simulink model "fermentation_dynamic_model_update"  (R2018a)
settings: Solver=VariableStepAuto  StartTime=0.0  StopTime=160  RelTol=1e-3
values from neighbouring files (symbols this model uses):
  ABV_lim = 0.0433    [fermentation_config_update.m]
  E_0 = 0    [fermentation_config_update.m]
  E_mol_mass = 0.04607    [fermentation_config_update.m]
  G_0 = 12.61/142.3*sum_sugars/0.180156    (= 104.992339972)    [fermentation_config_update.m]
  Kb = 10    [fermentation_config_update.m]
  Kd = 0    [fermentation_config_update.m]
  Ki = 0.1    [fermentation_config_update.m]
  Kp = 1.8    [fermentation_config_update.m]
  M_0 = 13.692/142.3*sum_sugars/0.3423    (= 60)    [fermentation_config_update.m]
  N = 0    [fermentation_config_update.m]
  N_0 = 116.205/143.2*sum_sugars/0.504437    (= 343.376857703)    [fermentation_config_update.m]
  p_KG = polyfit(T,K_G,1)    [fermentation_config_update.m]
  p_KiG = polyfit(T,Ki_G,1)    [fermentation_config_update.m]
  p_KiM = polyfit(T,Ki_M,1)    [fermentation_config_update.m]
  p_KM = polyfit(T,K_M,1)    [fermentation_config_update.m]
  p_KN = polyfit(T,K_N,1)    [fermentation_config_update.m]
  p_VG = polyfit(T,V_G,1)    [fermentation_config_update.m]
  p_VM = polyfit(T,V_M,1)    [fermentation_config_update.m]
  p_VN = polyfit(T,V_N,1)    [fermentation_config_update.m]
  R_EG = 1.92    [fermentation_config_update.m]
  R_EM = 3.84    [fermentation_config_update.m]
  R_EN = 5.76    [fermentation_config_update.m]
  R_XG = 0.134    [fermentation_config_update.m]
  R_XM = 0.268    [fermentation_config_update.m]
  R_XN = 0.402    [fermentation_config_update.m]
  T_0 = 12    [fermentation_config_update.m]
  T_c = 12    [fermentation_config_update.m]
  T_s = 12    [fermentation_config_update.m]
  X_0 = 200    [fermentation_config_update.m]
settings Model: Creator=Oscar  LastModifiedBy=Oscar

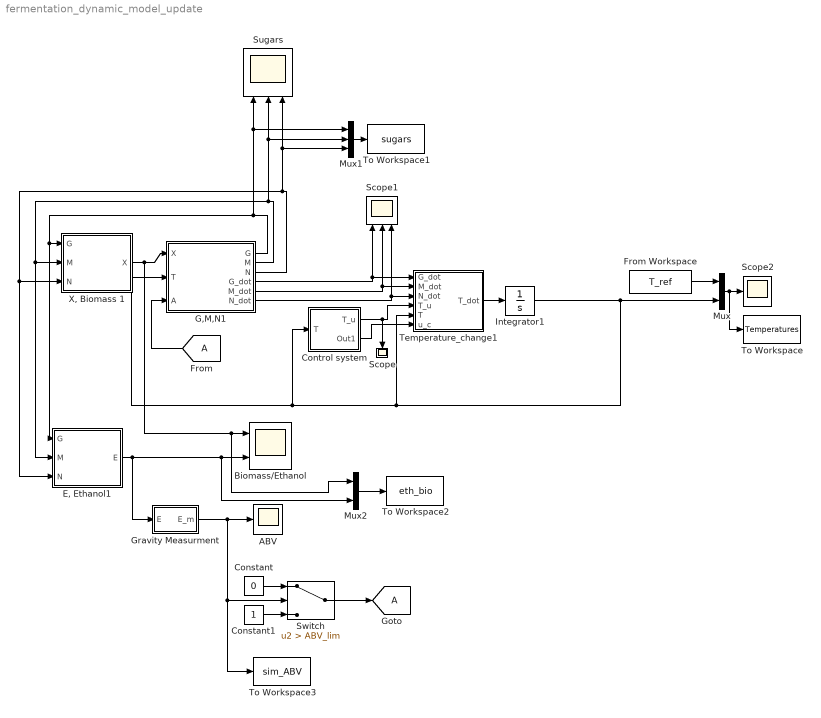
== system fermentation_dynamic_model_update ==
  ABV : Scope
  Biomass/Ethanol : Scope  NumInputPorts=2
  Constant : Constant  Value=0
  Constant1 : Constant
  Control system : Subsystem
  "E, Ethanol1" : Subsystem
  From Workspace : FromWorkspace  VariableName=T_ref  SampleTime=0
  G,M,N1 : Subsystem
  Gravity Measurment : Subsystem
  Integrator1 : Integrator  InitialCondition=T_0
  Mux : Mux  Inputs=2
  Mux1 : Mux  Inputs=3
  Mux2 : Mux  Inputs=2
  Scope : Scope
  Scope1 : Scope  NumInputPorts=3
  Scope2 : Scope
  Sugars : Scope  NumInputPorts=3
  Switch : Switch  Criteria=u2 > Threshold  Threshold=ABV_lim
  Temperature_change1 : MATLAB Function  TreatAsAtomicUnit=on
  To Workspace : ToWorkspace  VariableName=Temperatures  SaveFormat=Timeseries  SampleTime=-1
  To Workspace1 : ToWorkspace  VariableName=sugars  SaveFormat=Timeseries  SampleTime=-1
  To Workspace2 : ToWorkspace  VariableName=eth_bio  SaveFormat=Timeseries  SampleTime=-1
  To Workspace3 : ToWorkspace  VariableName=sim_ABV  SaveFormat=Timeseries  SampleTime=-1
  "X, Biomass 1" : Subsystem
  tag scope: A=global
  wires:
  From Workspace/1 -> Mux/1
  G,M,N1/2(M) -> "E, Ethanol1"/2(M), "X, Biomass 1"/2(M), Mux1/2, Sugars/2
  G,M,N1/6(N_dot) -> Scope1/3, Temperature_change1/3(N_dot)
  Mux1/1 -> To Workspace1/1
  Control system/1(T_u) -> Scope/1, Temperature_change1/4(T_u)
  Temperature_change1/1(T_dot) -> Integrator1/1
  G,M,N1/4(G_dot) -> Scope1/1, Temperature_change1/1(G_dot)
  Gravity Measurment/1("E_m ") -> To Workspace3/1, Switch/2, ABV/1
  G,M,N1/3(N) -> "X, Biomass 1"/3(N), "E, Ethanol1"/3(N), Mux1/3, Sugars/3
  "E, Ethanol1"/1(E) -> Gravity Measurment/1(E), Mux2/2, Biomass/Ethanol/2
  Mux/1 -> To Workspace/1, Scope2/1
  Control system/2(Out1) -> Temperature_change1/6(u_c)
  Mux2/1 -> To Workspace2/1
  "X, Biomass 1"/1(X) -> Mux2/1, Biomass/Ethanol/1, G,M,N1/1(X)
  G,M,N1/5(M_dot) -> Scope1/2, Temperature_change1/2(M_dot)
  G,M,N1/1(G) -> "E, Ethanol1"/1(G), "X, Biomass 1"/1(G), Mux1/1, Sugars/1
  Integrator1/1 -> Mux/2, G,M,N1/2("T "), Control system/1(T), Temperature_change1/5(T)
  [A] -> G,M,N1/3(A)
  Switch/1 -> [A]
  Constant/1 -> Switch/1
  Constant1/1 -> Switch/3

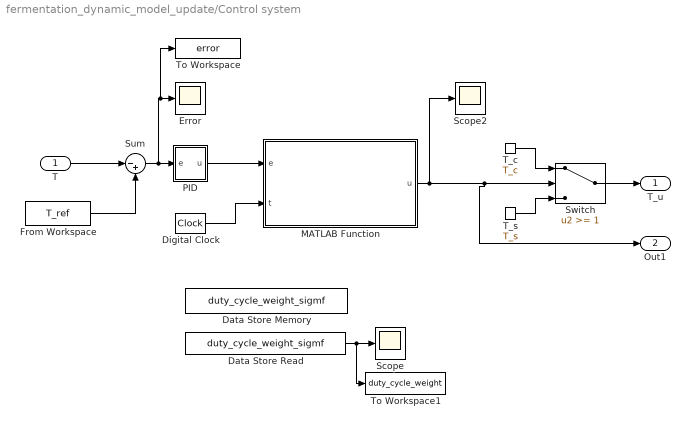
== system fermentation_dynamic_model_update/Control system ==
  T : Inport
  Data Store Memory : DataStoreMemory  DataStoreName=duty_cycle_weight_sigmf  ReadBeforeWriteMsg=warning  WriteAfterWriteMsg=warning  WriteAfterReadMsg=warning  ShowAdditionalParam=off  OutDataTypeStr=double
  Data Store Read : DataStoreRead  DataStoreName=duty_cycle_weight_sigmf
  Digital Clock : DigitalClock  SampleTime=0.001
  Error : Scope
  From Workspace : FromWorkspace  VariableName=T_ref  SampleTime=0
  MATLAB Function : MATLAB Function  TreatAsAtomicUnit=on
  PID : Subsystem
  Scope : Scope
  Scope2 : Scope
  Sum : Sum  Inputs=|-+
  Switch : Switch  Threshold=1
  T_c : Constant  Value=T_c
  T_s : Constant  Value=T_s
  To Workspace : ToWorkspace  VariableName=error  SaveFormat=Timeseries  SampleTime=-1
  To Workspace1 : ToWorkspace  VariableName=duty_cycle_weight  SaveFormat=Timeseries  SampleTime=-1
      settings: Save2DSignal=2-D array (concatenate along first dimension)
  T_u : Outport
  Out1 : Outport  Port=2
  wires:
  T/1 -> Sum/1
  T_c/1 -> Switch/1
  T_s/1 -> Switch/3
  Digital Clock/1 -> MATLAB Function/2(t)
  From Workspace/1 -> Sum/2
  Data Store Read/1 -> To Workspace1/1, Scope/1
  Switch/1 -> T_u/1
  MATLAB Function/1(u) -> Out1/1, Switch/2, Scope2/1
  Sum/1 -> PID/1(e), To Workspace/1, Error/1
  PID/1(u) -> MATLAB Function/1(e)

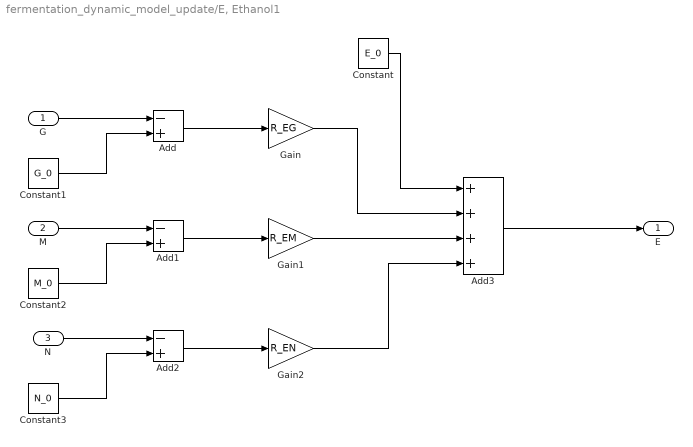
== system fermentation_dynamic_model_update/E, Ethanol1 ==
  G : Inport
  M : Inport  Port=2
  N : Inport  Port=3
  Add : Sum  Inputs=-+
  Add1 : Sum  Inputs=-+
  Add2 : Sum  Inputs=-+
  Add3 : Sum  Inputs=++++
  Constant : Constant  Value=E_0
  Constant1 : Constant  Value=G_0
  Constant2 : Constant  Value=M_0
  Constant3 : Constant  Value=N_0
  Gain : Gain  Gain=R_EG
  Gain1 : Gain  Gain=R_EM
  Gain2 : Gain  Gain=R_EN
  E : Outport
  wires:
  G/1 -> Add/1
  M/1 -> Add1/1
  N/1 -> Add2/1
  Constant3/1 -> Add2/2
  Constant2/1 -> Add1/2
  Constant1/1 -> Add/2
  Add/1 -> Gain/1
  Add1/1 -> Gain1/1
  Add2/1 -> Gain2/1
  Add3/1 -> E/1
  Constant/1 -> Add3/1
  Gain/1 -> Add3/2
  Gain1/1 -> Add3/3
  Gain2/1 -> Add3/4

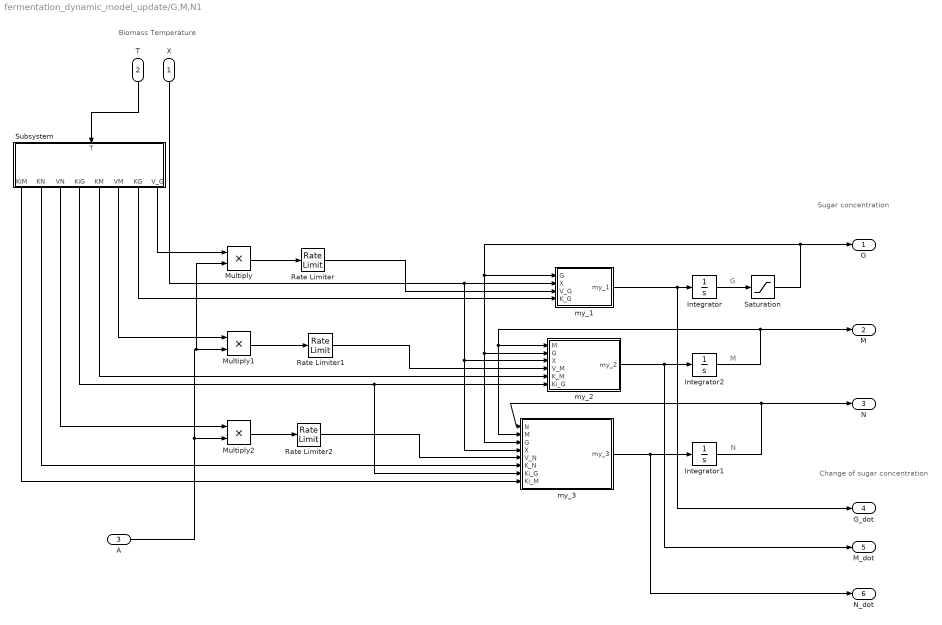
== system fermentation_dynamic_model_update/G,M,N1 ==
  note: Change of sugar
      | concentration
  note: Sugar concentration
  note: Biomass
      | Temperature
  note: N
  note: M
  note: G
  X : Inport
  "T " : Inport  Port=2
  A : Inport  Port=3
  Integrator : Integrator  InitialCondition=G_0
  Integrator1 : Integrator  InitialCondition=N_0
  Integrator2 : Integrator  InitialCondition=M_0
  Multiply : Product
  Multiply1 : Product
  Multiply2 : Product
  Rate Limiter : RateLimiter  RisingSlewLimit=0.0001  FallingSlewLimit=-0.00001  SampleTimeMode=inherited
  Rate Limiter1 : RateLimiter  RisingSlewLimit=0.0001  FallingSlewLimit=-0.00001  SampleTimeMode=inherited
  Rate Limiter2 : RateLimiter  RisingSlewLimit=0.0001  FallingSlewLimit=-0.00001  SampleTimeMode=inherited
  Saturation : Saturate  UpperLimit=inf  LowerLimit=0
  Subsystem : Subsystem
  my_1 : MATLAB Function  TreatAsAtomicUnit=on
  my_2 : MATLAB Function  TreatAsAtomicUnit=on
  my_3 : MATLAB Function  TreatAsAtomicUnit=on
  G : Outport
  M : Outport  Port=2
  N : Outport  Port=3
  G_dot : Outport  Port=4
  M_dot : Outport  Port=5
  N_dot : Outport  Port=6
  wires:
  Integrator/1 -> Saturation/1
  Integrator1/1 -> my_3/1(N), N/1
  Integrator2/1 -> my_3/2(M), my_2/1(M), M/1
  X/1 -> my_3/4(X), my_2/3(X), my_1/2(X)
  "T "/1 -> Subsystem/1(T)
  Subsystem/1(KiM) -> my_3/8(Ki_M)
  Subsystem/4(KiG) -> my_2/6(Ki_G), my_3/7(Ki_G)
  Subsystem/2(KN) -> my_3/6(K_N)
  Subsystem/5(KM) -> my_2/5(K_M)
  Subsystem/7(KG) -> my_1/4(K_G)
  Saturation/1 -> G/1, my_1/1(G), my_2/2(G), my_3/3(G)
  Multiply/1 -> Rate Limiter/1
  Multiply1/1 -> Rate Limiter1/1
  Multiply2/1 -> Rate Limiter2/1
  A/1 -> Multiply/2, Multiply1/2, Multiply2/2
  Subsystem/8(V_G) -> Multiply/1
  Subsystem/6(VM) -> Multiply1/1
  Subsystem/3(VN) -> Multiply2/1
  my_1/1(my_1) -> G_dot/1, Integrator/1
  my_3/1(my_3) -> N_dot/1, Integrator1/1
  my_2/1(my_2) -> M_dot/1, Integrator2/1
  Rate Limiter/1 -> my_1/3(V_G)
  Rate Limiter1/1 -> my_2/4(V_M)
  Rate Limiter2/1 -> my_3/5(V_N)

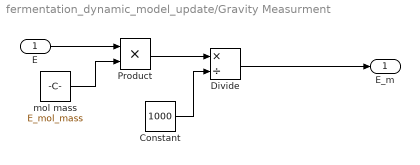
== system fermentation_dynamic_model_update/Gravity Measurment ==
  E : Inport
  Constant : Constant  Value=1000
  Divide : Product  Inputs=*/
  Product : Product
  mol mass : Constant  Value=E_mol_mass
  "E_m " : Outport
  wires:
  E/1 -> Product/1
  mol mass/1 -> Product/2
  Product/1 -> Divide/1
  Constant/1 -> Divide/2
  Divide/1 -> "E_m "/1

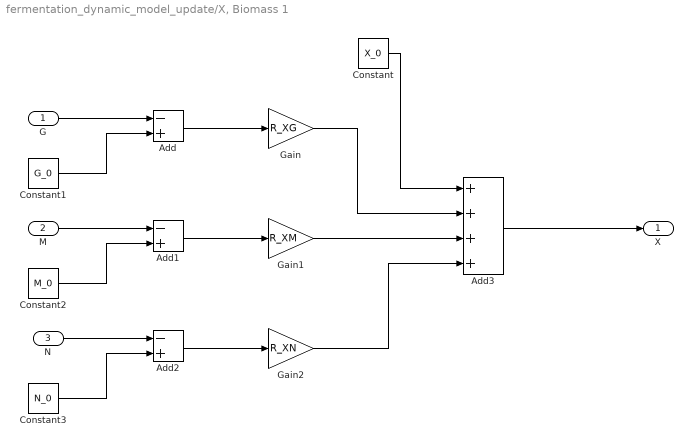
== system fermentation_dynamic_model_update/X, Biomass 1 ==
  G : Inport
  M : Inport  Port=2
  N : Inport  Port=3
  Add : Sum  Inputs=-+
  Add1 : Sum  Inputs=-+
  Add2 : Sum  Inputs=-+
  Add3 : Sum  Inputs=++++
  Constant : Constant  Value=X_0
  Constant1 : Constant  Value=G_0
  Constant2 : Constant  Value=M_0
  Constant3 : Constant  Value=N_0
  Gain : Gain  Gain=R_XG
  Gain1 : Gain  Gain=R_XM
  Gain2 : Gain  Gain=R_XN
  X : Outport
  wires:
  G/1 -> Add/1
  M/1 -> Add1/1
  N/1 -> Add2/1
  Constant3/1 -> Add2/2
  Constant2/1 -> Add1/2
  Constant1/1 -> Add/2
  Add/1 -> Gain/1
  Add1/1 -> Gain1/1
  Add2/1 -> Gain2/1
  Add3/1 -> X/1
  Constant/1 -> Add3/1
  Gain/1 -> Add3/2
  Gain1/1 -> Add3/3
  Gain2/1 -> Add3/4

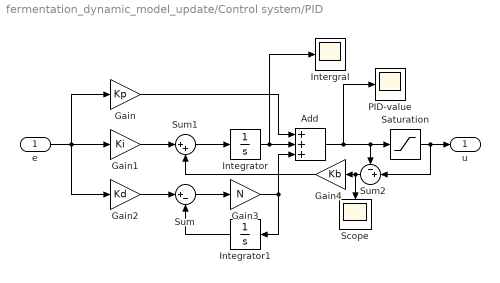
== system fermentation_dynamic_model_update/Control system/PID ==
  e : Inport
  Add : Sum  Inputs=3
  Gain : Gain  Gain=Kp
  Gain1 : Gain  Gain=Ki
  Gain2 : Gain  Gain=Kd
  Gain3 : Gain  Gain=N
  Gain4 : Gain  Gain=Kb
  Integrator : Integrator
  Integrator1 : Integrator
  "Intergral " : Scope
  PID-value : Scope
  Saturation : Saturate  UpperLimit=20  LowerLimit=-10
  Scope : Scope
  Sum : Sum  Inputs=|+-
  Sum1 : Sum  Inputs=|++
  Sum2 : Sum  Inputs=-+|
  u : Outport
  wires:
  Add/1 -> PID-value/1, Saturation/1, Sum2/1
  e/1 -> Gain/1, Gain2/1, Gain1/1
  Gain/1 -> Add/1
  Gain2/1 -> Sum/1
  Sum/1 -> Gain3/1
  Integrator1/1 -> Sum/2
  Gain3/1 -> Add/3, Integrator1/1
  Integrator/1 -> "Intergral "/1, Add/2
  Sum1/1 -> Integrator/1
  Gain1/1 -> Sum1/1
  Gain4/1 -> Sum1/2
  Sum2/1 -> Gain4/1, Scope/1
  Saturation/1 -> Sum2/2, u/1

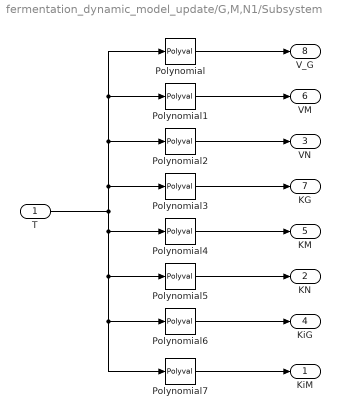
== system fermentation_dynamic_model_update/G,M,N1/Subsystem ==
  T : Inport
  Polynomial : Polyval  Coefs=p_VG
  Polynomial1 : Polyval  Coefs=p_VM
  Polynomial2 : Polyval  Coefs=p_VN
  Polynomial3 : Polyval  Coefs=p_KG
  Polynomial4 : Polyval  Coefs=p_KM
  Polynomial5 : Polyval  Coefs=p_KN
  Polynomial6 : Polyval  Coefs=p_KiG
  Polynomial7 : Polyval  Coefs=p_KiM
  KiM : Outport
  KN : Outport  Port=2
  VN : Outport  Port=3
  KiG : Outport  Port=4
  KM : Outport  Port=5
  VM : Outport  Port=6
  KG : Outport  Port=7
  V_G : Outport  Port=8
  wires:
  Polynomial/1 -> V_G/1
  Polynomial1/1 -> VM/1
  Polynomial2/1 -> VN/1
  Polynomial3/1 -> KG/1
  Polynomial4/1 -> KM/1
  Polynomial5/1 -> KN/1
  Polynomial6/1 -> KiG/1
  Polynomial7/1 -> KiM/1
  T/1 -> Polynomial2/1, Polynomial1/1, Polynomial/1, Polynomial3/1, Polynomial4/1, Polynomial7/1, Polynomial6/1, Polynomial5/1

== matlab function fermentation_dynamic_model_update/Control system/MATLAB Function ==
  settings: updateMethod=DISCRETE
  data: e input; u output; t input; duty_cycle_weight_sigmf data_store_memory
function u  = duty_cycle(e,t)
global  duty_cycle_weight_sigmf
% Slope of the sigmoid function
sig_slope = 3;
% Point of 1/2 output from the sigmoid function
sig_half= 0.45; 
% Duty time which gets divided to an active and an inactive phase
duty_cycle_time = 0.25;
% The modulus of the current time of the cycle time corresponds to
% percentage of the current cycle
t_in_cycle=mod(t,duty_cycle_time);

% Approx steady state active phase
if t_in_cycle ==0
duty_cycle_weight_sigmf = sigmf(e,[sig_slope,sig_half]);
end

if  t_in_cycle/duty_cycle_time > duty_cycle_weight_sigmf
    u=1;
else
    u=0;
end

== matlab function fermentation_dynamic_model_update/G,M,N1/my_1 ==
  data: G input; my_1 output; X input; V_G input; K_G input
function my_1 = fcn(G,X, V_G, K_G)
%#codegen

my_1 = -(V_G*G)/(K_G + G)*X;

== matlab function fermentation_dynamic_model_update/G,M,N1/my_2 ==
  data: M input; G input; my_2 output; X input; V_M input; K_M input; Ki_G input
function my_2 = fcn(M,G,X, V_M, K_M, Ki_G)
%#codegen

my_2 = -((V_M*M)/(K_M + M)*(Ki_G/(Ki_G + G)))*X;

== matlab function fermentation_dynamic_model_update/G,M,N1/my_3 ==
  data: N input; M input; G input; my_3 output; X input; V_N input; K_N input; Ki_G input; Ki_M input
function my_3 = fcn(N,M,G,X, V_N, K_N, Ki_G, Ki_M)
%#codegen



my_3 = -((V_N*N)/(K_N + N)*Ki_M/(Ki_M + M)*Ki_G/(Ki_G + G))*X;

== matlab function fermentation_dynamic_model_update/Temperature_change1 ==
  data: G_dot input; T_dot output; M_dot input; N_dot input; T_u input; T input; u_c input
function T_dot = fcn(G_dot,M_dot,N_dot,T_u,T,u_c)
%#codegen

rho = 1.06;
Cp = 4000;

DH_RG = -91.2;
DH_RM = -226.3;
DH_RN = -361.3;

U = 23000;
Area = 0.188;
V = 1;

if u_c
u = 1000;
else
    u=50;
end

T_dot = 1/(rho*Cp)*(DH_RG*G_dot + DH_RM*M_dot + DH_RN*N_dot - u*(T - T_u));
